simulink model "lab_1_f"  (R2025b)
settings: Solver=VariableStepAuto  StartTime=0.0  StopTime=10.0  RelTol=1e-3
values from neighbouring files (symbols this model uses):
  k1 = (tau * (omega^2))/kp    [lab_1.m]
  kp = 35    [lab_1.m]
  tau = 1/(2 * zeta * omega)    [lab_1.m]
settings Model: Creator=ishraqanwar  LastModifiedBy=sengu

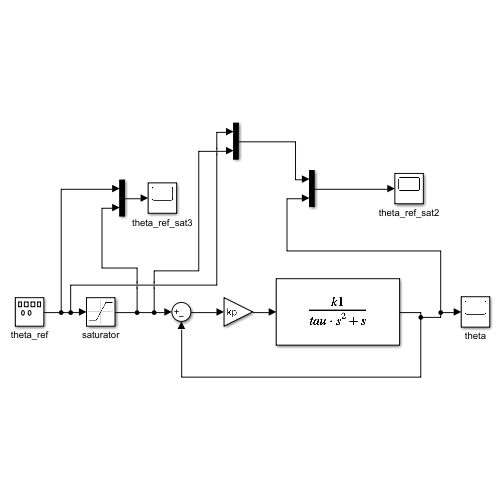
[thumbnail: Simulink's stored preview of the top-level diagram]
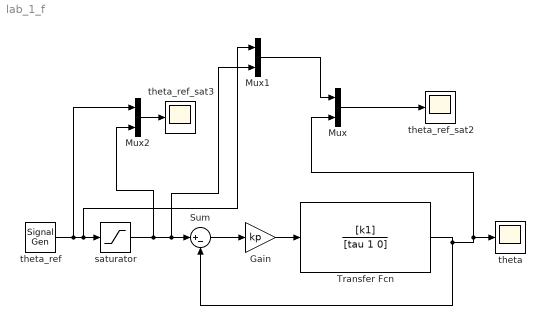
== system lab_1_f ==
  Gain : Gain  Gain=kp
  Mux : Mux  Inputs=2
  Mux1 : Mux  Inputs=2
  Mux2 : Mux  Inputs=2
  Sum : Sum  Inputs=|+-
  Transfer Fcn : TransferFcn  Numerator=[k1]  Denominator=[tau 1 0]
  saturator : Saturate  UpperLimit=0.7  LowerLimit=-0.7
  theta : Scope
      settings: ActiveDisplayYMinimum=-1.39899  ActiveDisplayYMaximum=1.3974
  theta_ref : SignalGenerator  WaveForm=square  Amplitude=1.0  Frequency=0.5
  theta_ref_sat2 : Scope
      settings: ActiveDisplayYMinimum=-1  ActiveDisplayYMaximum=1  DataLoggingVariableName=ScopeData3
  theta_ref_sat3 : Scope
      settings: ActiveDisplayYMinimum=-1.25  ActiveDisplayYMaximum=1.25  DataLoggingVariableName=ScopeData4
  wires:
  saturator/1 -> Mux2/2, Mux1/2, Sum/1
  Sum/1 -> Gain/1
  Gain/1 -> Transfer Fcn/1
  Transfer Fcn/1 -> Sum/2, Mux/2, theta/1
  theta_ref/1 -> Mux2/1, Mux1/1, saturator/1
  Mux/1 -> theta_ref_sat2/1
  Mux1/1 -> Mux/1
  Mux2/1 -> theta_ref_sat3/1
